simulink model "closedLoopModel"  (R2026a)
settings: Solver=FixedStepDiscrete  StopTime=8000  FixedStep=1
model workspace (MAT data in the model file):
  I_charge = 2.5
  OCV_LUT = [3.22368449776 3.22907500736 3.23446551696 3.23985602656 3.42160174835 3.48094057268 3.53092121085 3.57607683205 3.6153857338 3.65272792805 3.69678052748 3.75248114251 3.8047311296 3.85856315106 3.90906765508 3.95653146496 4.0176577851 4.07696384653 4.10136153414 4.13216876748 4.19091545645]
  Q_Ah = 2.65479463269
  R0 = 0.0211720623698
  R1 = 0.0309885930255
  SOC0 = 0.85
  SOC_bp = [0 0.05 0.1 0.15 0.2 0.25 0.3 0.35 0.4 0.45 0.5 0.55 0.6 0.65 0.7 0.75 0.8 0.85 0.9 0.95 1]
  T_amb = 25
  Xmax = [4.23207255751; 5.99961; 26.81543]
  Xmin = [2.79645479834; -18.0971537397; -10.3047309401]
  aRC = 0.983471453822
  driveProfile = [-0.7 -0.7 -0.7 -0.7 -0.7 -0.7 -0.7 -0.7 -0.7 -0.7 -0.7 -0.7 ... (400 elements, 1x400)]
undefined symbols (not defined in the file): DiscIntNeverNeededParam
libraries: simulink x2, deeplib x1
settings Model: PacingRate=200  Creator=KoayXianCong  LastModifiedBy=KoayXianCong

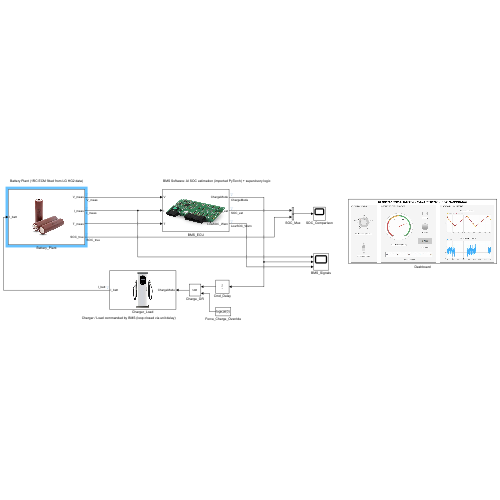
[thumbnail: Simulink's stored preview of the top-level diagram]
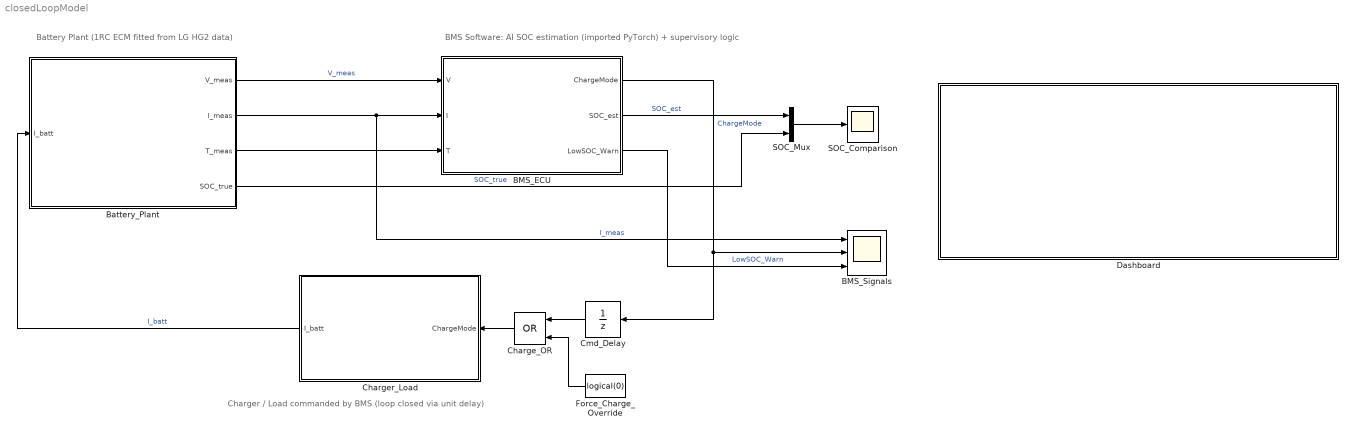
== system closedLoopModel ==
  note: Battery Plant (1RC ECM fitted from LG HG2 data)
  note: BMS Software: AI SOC estimation (imported PyTorch) + supervisory logic
  note: Charger / Load commanded by BMS (loop closed via unit delay)
  BMS_ECU : Subsystem
      mask Display: image('bms_ecu.png');
  BMS_Signals : Scope  NumInputPorts=3
  Battery_Plant : Subsystem
      mask Display: image('battery.jpg');
  Charge_OR : Logic  Operator=OR
  Charger_Load : Subsystem
      mask Display: image('charger.png');
  Cmd_Delay : UnitDelay
  Dashboard : Subsystem
      mask Display: image('dashboard.jpg');
  Force_Charge_Override : Constant  Value=logical(0)  OutDataTypeStr=boolean
  SOC_Comparison : Scope
  SOC_Mux : Mux  Inputs=2
  wires:
  Battery_Plant/1(V_meas) -> BMS_ECU/1(V)  "V_meas"
  Battery_Plant/2(I_meas) -> BMS_Signals/1, BMS_ECU/2(I)  "I_meas"
  Battery_Plant/3(T_meas) -> BMS_ECU/3(T)
  BMS_ECU/1(ChargeMode) -> Cmd_Delay/1, BMS_Signals/2  "ChargeMode"
  Cmd_Delay/1 -> Charge_OR/1
  Force_Charge_Override/1 -> Charge_OR/2
  Charge_OR/1 -> Charger_Load/1(ChargeMode)
  Charger_Load/1(I_batt) -> Battery_Plant/1(I_batt)  "I_batt"
  Battery_Plant/4(SOC_true) -> SOC_Mux/2  "SOC_true"
  BMS_ECU/2(SOC_est) -> SOC_Mux/1  "SOC_est"
  SOC_Mux/1 -> SOC_Comparison/1
  BMS_ECU/3(LowSOC_Warn) -> BMS_Signals/3  "LowSOC_Warn"

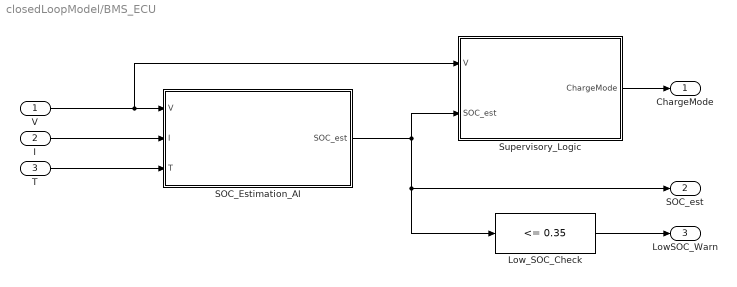
== system closedLoopModel/BMS_ECU ==
  V : Inport
  I : Inport  Port=2
  T : Inport  Port=3
  Low_SOC_Check : simulink/Logic and Bit Operations/Compare To Constant  relop=<=  const=0.35  OutDataTypeStr=boolean
  SOC_Estimation_AI : Subsystem
      mask Display: image('dnn.png');
  Supervisory_Logic : Stateflow chart  TreatAsAtomicUnit=on
      settings: PortSchema="{\"entries\":[{\"content\":{\"sides\":[{\"content\":{\"connectorIds\":[\"In2\",\"In1\"]},\"type\":\"ConnectorPlacement.EquallySpacedRectSide\",\"uuid\":\"081fad27-0f30-48d6-a20d-5f64585075c8\"},{\"content\":{\"connectorIds\":[\"Out1\"],\"side\":\"RIGHT\"},\"type\":\"ConnectorPlacement.EquallySpacedRectSide\",\"uuid\":\"4c761981-9626-4ab6-9fe4-cdd2589e22a3\"},{\"content\":{\"side\":\"TOP\"},\"type\":\"ConnectorPlacement.EquallySpacedRectSide\",\"uuid\":\"47498760-84fa-45ce-bcf4-c45055da7767\"}]},\"type\":\"ConnectorPlacement.EquallySpacedConnector\",\"uuid\":\"c8b4ca25-75c7-455a-83f9-bfdc8e44a844\"}],\"packageUris\":[\"http://schema.mathworks.com/mf0/Connector/R2020b\"],\"version\":\"1.0\"}"
  ChargeMode : Outport
  SOC_est : Outport  Port=2
  LowSOC_Warn : Outport  Port=3
  wires:
  V/1 -> SOC_Estimation_AI/1(V), Supervisory_Logic/2(V)
  I/1 -> SOC_Estimation_AI/2(I)
  T/1 -> SOC_Estimation_AI/3(T)
  SOC_Estimation_AI/1(SOC_est) -> Low_SOC_Check/1, SOC_est/1, Supervisory_Logic/1(SOC_est)
  Supervisory_Logic/1(ChargeMode) -> ChargeMode/1
  Low_SOC_Check/1 -> LowSOC_Warn/1

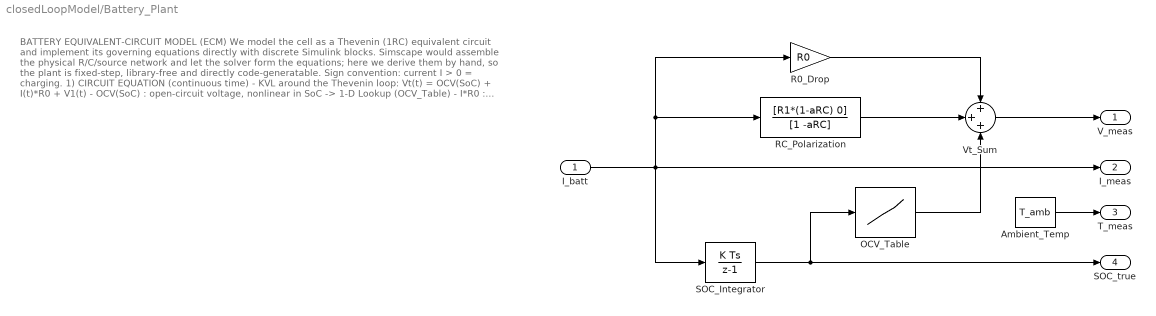
== system closedLoopModel/Battery_Plant ==
  note: BATTERY EQUIVALENT-CIRCUIT MODEL (ECM)
      |
      | We model the cell as a Thevenin (1RC) equivalent circuit and implement its governing
      | equations directly with discrete Simulink blocks. Simscape would assemble the physical
      | R/C/source network and let the solver form the equations; here we derive them by hand,
      | so the plant is fixed-step, library-free and directly code-generatable.
      | Sign convention: current I > 0 = charging.
      |
      | 1) CIRCUIT EQUATION (continuous time)  -  KVL around the Thevenin loop:
      |        Vt(t) = OCV(SoC) + I(t)*R0 + V1(t)
      |    - OCV(SoC) : open-circuit voltage, nonlinear in SoC      -> 1-D Lookup (OCV_Table)
      |    - I*R0     : instantaneous ohmic drop across series R0   -> Gain (R0_Drop)
      |    - V1       : voltage across the R1||C1 branch            -> see (2)
      |
      | 2) RC BRANCH DYNAMICS  -  KCL at the R1||C1 node (cap. current + resistor current = I):
      |        C1*dV1/dt + V1/R1 = I
      |    =>  dV1/dt = -V1/tau + (R1/tau)*I ,      tau = R1*C1
      |    Step response (I constant):  V1(t) = R1*I*(1 - exp(-t/tau))
      |    -> R1 sets the steady-state drop, tau = R1*C1 sets how fast it settles.
      |
      | 3) EXACT DISCRETIZATION (zero-order hold, sample time Ts = 1 s)
      |    Integrating the 1st-order ODE over one step with I held constant:
      |        V1[k] = a*V1[k-1] + R1*(1-a)*I[k] ,      a = exp(-Ts/tau)
      |    As a discrete transfer function:
      |        V1(z)/I(z) = R1*(1-a) / (1 - a*z^-1)
      |    -> Discrete Transfer Fcn:  num = [R1*(1-a)  0],  den = [1  -a]   (a = aRC in the model)
      |
      | 4) STATE OF CHARGE  -  Coulomb counting (charge balance):
      |        dSoC/dt = I / (3600*Q)        (Q in Ah, I in A, 3600 s/h)
      |    Forward-Euler discrete form:
      |        SoC[k] = SoC[k-1] + Ts*I[k] / (3600*Q)
      |    -> Discrete-Time Integrator, gain 1/(3600*Q), saturated to [0,1].
      |       Its output is the TRUE SoC used to score the AI estimate.
      |
      | Parameters Q, OCV(.), R0, R1, tau are least-squares fitted from LG HG2 cell data.
      | Temperature is held at 25 deg C in this demo.
  I_batt : Inport
  Ambient_Temp : Constant  Value=T_amb
  OCV_Table : Lookup_n-D  NumberOfTableDimensions=1  BreakpointsForDimension1=SOC_bp  Table=OCV_LUT  InternalRulePriority=Speed  RndMeth=Simplest
  R0_Drop : Gain  Gain=R0
  RC_Polarization : DiscreteTransferFcn  Numerator=[R1*(1-aRC) 0]  Denominator=[1 -aRC]  SampleTime=1
  SOC_Integrator : DiscreteIntegrator  gainval=1/(3600*Q_Ah)  InitialCondition=SOC0  LimitOutput=on  UpperSaturationLimit=1  LowerSaturationLimit=0  ICPrevOutput=DiscIntNeverNeededParam  ICPrevScaledInput=DiscIntNeverNeededParam
  Vt_Sum : Sum  Inputs=+++
  V_meas : Outport
  I_meas : Outport  Port=2
  T_meas : Outport  Port=3
  SOC_true : Outport  Port=4
  wires:
  I_batt/1 -> RC_Polarization/1, R0_Drop/1, SOC_Integrator/1, I_meas/1
  SOC_Integrator/1 -> SOC_true/1, OCV_Table/1
  OCV_Table/1 -> Vt_Sum/3
  RC_Polarization/1 -> Vt_Sum/2
  R0_Drop/1 -> Vt_Sum/1
  Vt_Sum/1 -> V_meas/1
  Ambient_Temp/1 -> T_meas/1

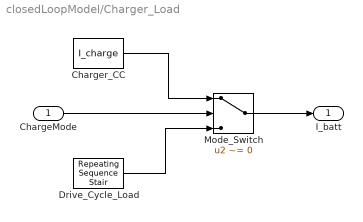
== system closedLoopModel/Charger_Load ==
  ChargeMode : Inport
  Charger_CC : Constant  Value=I_charge
  Drive_Cycle_Load : simulink/Sources/Repeating Sequence Stair  OutValues=driveProfile  tsamp=1  OutMin=[]  OutMax=[]  OutDataTypeStr=double  OutputDataTypeScalingMode=double  OutDataType=fixdt(0,8)  ConRadixGroup=Best Precision: Vector-wise  OutScaling=2^-12
  Mode_Switch : Switch  Criteria=u2 ~= 0
  I_batt : Outport
  wires:
  Charger_CC/1 -> Mode_Switch/1
  ChargeMode/1 -> Mode_Switch/2
  Drive_Cycle_Load/1 -> Mode_Switch/3
  Mode_Switch/1 -> I_batt/1

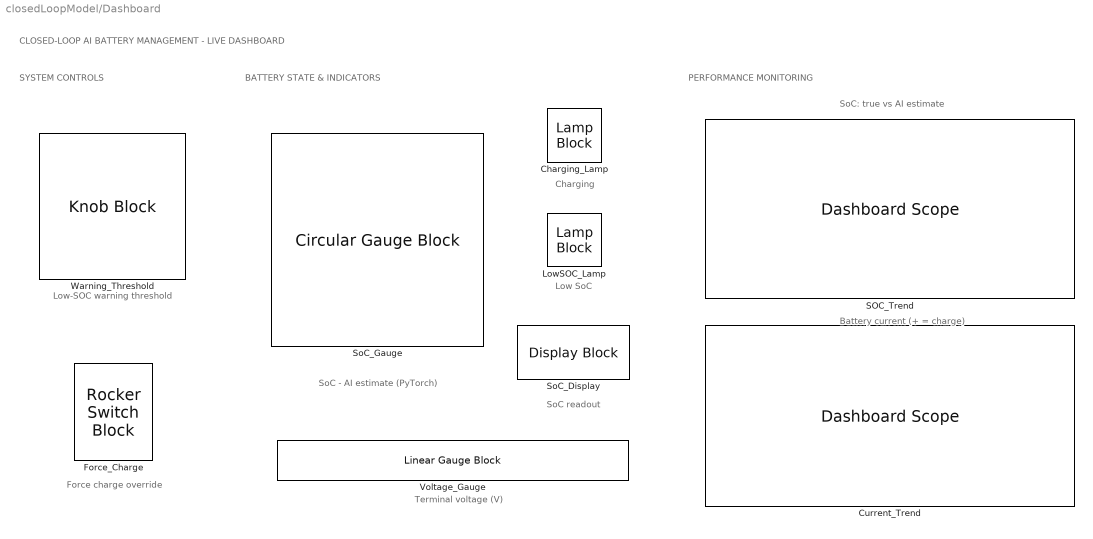
== system closedLoopModel/Dashboard ==
  note: CLOSED-LOOP AI BATTERY MANAGEMENT - LIVE DASHBOARD
  note: SYSTEM CONTROLS
  note: BATTERY STATE & INDICATORS
  note: PERFORMANCE MONITORING
  note: Low-SOC warning threshold
  note: Force charge override
  note: SoC - AI estimate (PyTorch)
  note: Terminal voltage (V)
  note: Charging
  note: Low SoC
  note: SoC readout
  note: SoC: true vs AI estimate
  note: Battery current (+ = charge)
  Charging_Lamp : LampBlock  LabelPosition=Hide  DefaultColor=[192.0, 192.0, 192.0]  Icon=Battery
  Current_Trend : DashboardScope  TimeSpan=8000  Ymin=-10  Ymax=5  ScaleAtStop=off  FontColor=[0.0, 0.0, 0.0]
  Force_Charge : RockerSwitchBlock  LabelPosition=Hide
  LowSOC_Lamp : LampBlock  LabelPosition=Hide  DefaultColor=[192.0, 192.0, 192.0]
  SOC_Trend : DashboardScope  TimeSpan=8000  Ymin=0  Ymax=1  ScaleAtStop=off  FontColor=[0.0, 0.0, 0.0]
  SoC_Display : DisplayBlock  LabelPosition=Hide  Transparency=1  GridColor=[0.502, 0.502, 0.502]
  SoC_Gauge : CircularGaugeBlock  LabelPosition=Hide  ScaleMax=1  TickInterval=0.2  FontColor=[0.0, 0.0, 0.0]
  Voltage_Gauge : LinearGaugeBlock  LabelPosition=Hide  ScaleMin=2.8  ScaleMax=4.4  TickInterval=0.4  FontColor=[0.0, 0.0, 0.0]
  Warning_Threshold : KnobBlock  LabelPosition=Hide  ScaleMax=1  TickInterval=0.25

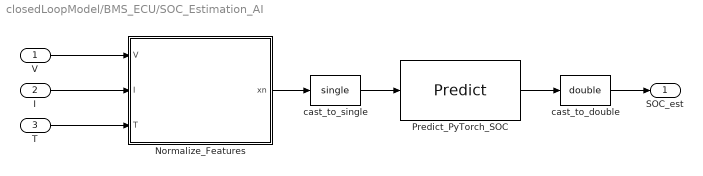
== system closedLoopModel/BMS_ECU/SOC_Estimation_AI ==
  V : Inport
  I : Inport  Port=2
  T : Inport  Port=3
  Normalize_Features : MATLAB Function  TreatAsAtomicUnit=on
  Predict_PyTorch_SOC : deeplib/Predict  Network=Network from MAT-file  NetworkFunction=squeezenet  NetworkFilePath=netPyTorchMLP.mat  MiniBatchSize=128  SimulateUsing=Auto mode  InputDataFormats={'input_1', 'UU';}  Predictions=on  Activations={}  ForceInterpretedSim=off  EnableDLNetwork=on  LastKnownNetworkFilePath='netPyTorchMLP.mat'  LastKnownNetworkTimeStamp=740142.380682870396412909030914306640625
  cast_to_double : DataTypeConversion  OutDataTypeStr=double
  cast_to_single : DataTypeConversion  OutDataTypeStr=single
  SOC_est : Outport
  wires:
  V/1 -> Normalize_Features/1(V)
  I/1 -> Normalize_Features/2(I)
  T/1 -> Normalize_Features/3(T)
  Normalize_Features/1(xn) -> cast_to_single/1
  cast_to_single/1 -> Predict_PyTorch_SOC/1
  Predict_PyTorch_SOC/1 -> cast_to_double/1
  cast_to_double/1 -> SOC_est/1

== matlab function closedLoopModel/BMS_ECU/SOC_Estimation_AI/Normalize_Features ==
  data: V input; xn output; I input; T input; Xmin parameter; Xmax parameter
function xn = normalizeFeatures(V, I, T, Xmin, Xmax)
% Feature preparation for the imported PyTorch SOC network.
% Mirrors BatteryManagementSystem/SOC_Estimation_NN Arrange_Data/Normalize:
% min/max scaling plus trailing moving averages of voltage and current.
W = 500;  % window used when the LG HG2 training data was prepared
persistent vBuf iBuf n
if isempty(n)
    vBuf = zeros(1,W); iBuf = zeros(1,W); n = 0;
end
vn = (V - Xmin(1))/(Xmax(1) - Xmin(1));
in_ = (I - Xmin(2))/(Xmax(2) - Xmin(2));
tn = (T - Xmin(3))/(Xmax(3) - Xmin(3));
vBuf = [vn, vBuf(1:W-1)];
iBuf = [in_, iBuf(1:W-1)];
n = min(n+1, W);
avgV = sum(vBuf)/n;   % growing window until buffer is full
avgI = sum(iBuf)/n;
xn = [vn; in_; tn; avgV; avgI];

== stateflow chart closedLoopModel/BMS_ECU/Supervisory_Logic ==
  state Drive
    entry:
    ChargeMode = false;
  state Charge
    entry:
    ChargeMode = true;
  (default) -> Drive
  Drive -> Charge : [SOC_est <= 0.30]
  Charge -> Drive : [SOC_est >= 0.90 || V >= 4.28]
  data: SOC_est input; V input; ChargeMode output boolean
